simulink model "robot_linear_model"  (R2024b)
settings: Solver=VariableStepAuto  StartTime=0.0  StopTime=10.0  RelTol=1e-3
model workspace (MAT data in the model file):
  pitchd = Simulink.Parameter
  pitchd.Value = 1
  pitchd.Complexity = 'real'
  pitchd.Dimensions = [1 1]
  pitchd.DataType = 'auto'
  yawd = Simulink.Parameter
  yawd.Value = 1
  yawd.Complexity = 'real'
  yawd.Dimensions = [1 1]
  yawd.DataType = 'auto'
values from neighbouring files (symbols this model uses):
  A = [0   1.0000        0        0 ... (first row only)    [invgui.m]    (also in p1.m = 14; p2.m = 14; robot.m = [0 1 0 0; robot_cascade.m = [ 0, 1, 0, 0)
  B = [0; 1.8182; 0; 4.5455]    [invgui.m]    (also in p1.m = 18; p2.m = 18; robot.m = B ./ R; robot_cascade.m = B ./ r_wheel)
  C_xt = eye(4)    [robot.m]    (also in robot_cascade.m; robot_linear.m; robot_lqr.m)
  D_xt = [0;0;0;0]    [robot.m]    (also in robot_cascade.m; robot_linear.m; robot_lqr.m)
  Km = 0.212207    [robot.m]    (also in robot_cascade.m = 16.1290322581; robot_linear.m; robot_lqr.m)
  n = 18.75    [robot.m]    (also in robot_cascade.m; robot_linear.m; robot_lqr.m)
  r_wheel = 0.04    [robot_cascade.m]    (also in robot_linear.m; robot_lqr.m)
libraries: cstblocks x8, slctrl_autotuning x1, slpidlib x1
settings Model: Creator=cosr3  LastModifiedBy=cosr3

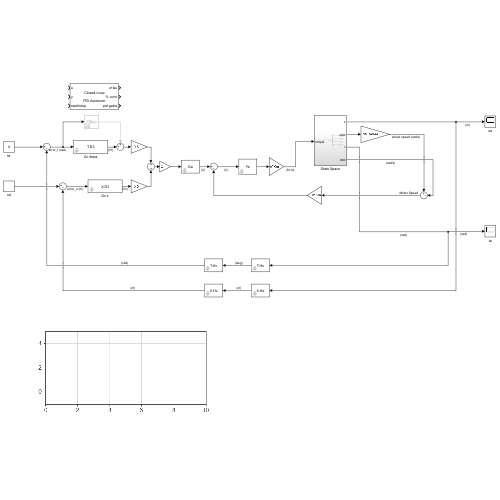
[thumbnail: Simulink's stored preview of the top-level diagram]
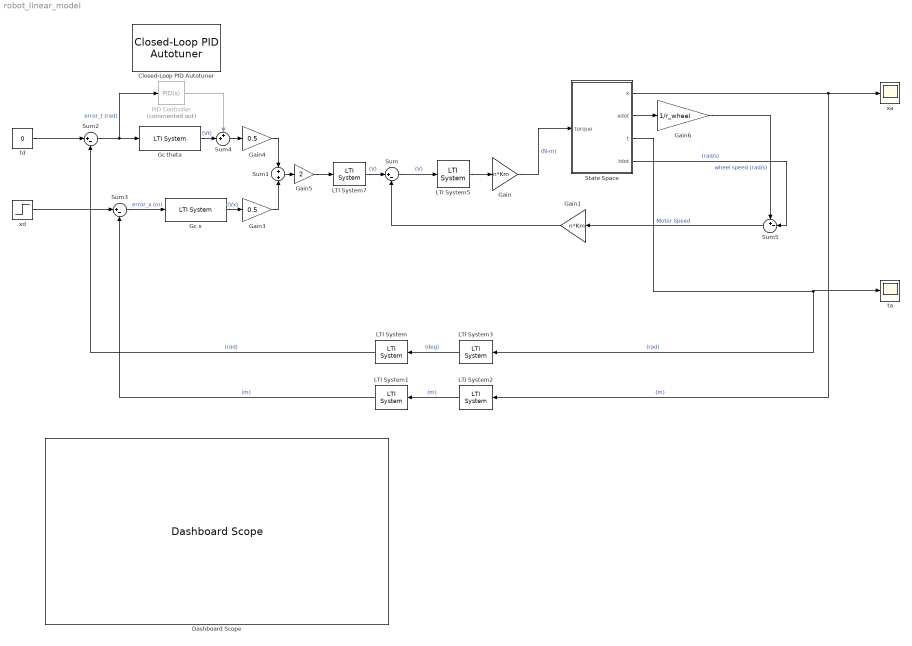
== system robot_linear_model ==
  Closed-Loop PID Autotuner : slctrl_autotuning/Closed-Loop PID Autotuner  PIDType=PI  PIDForm=Parallel  TimeDomain=discrete-time  DiscreteTs=0.1  TuningTs=0.2  UseTuningTs=off  IntegratorFormula=Forward Euler  FilterFormula=Forward Euler  ContinuousTs=0.02  Bandwidth=1  UseExternalWC=off  TargetPM=60  UseExternalPM=off  UseExternalAchievedPM=off  ExperimentMode=Superposition  PlantType=Stable  PlantSign=Positive  AmpSine=1  UseExternalAmpSine=off  UseExternalFRD=off  UseExternalU0=off  UseCompanion=off  NotDeployTuningModule=off  UsePLCCoder=off  OutputMode=control action + perturbation  BlockDataType=double  UseConnectedPID=on  blockpath=[]  tunedP=0  tunedI=0  tunedD=0  tunedN=100  tunedPM=0  EstimationWindowSize=3  UseExternalTuningParams=off  SingleMultiRateVariant=SingleSamplingRate  NumEstimationPeriods=4  NumSettlingPeriods=2  NumOfPRBSPeriod=1  PRBSSignalOrder=12  ExperimentModeVariant=VariantSuperimposed  OutputChoice=VariantCandD  ConvergenceCalcVariant=ConvSuperpositionPRBSVariant
      settings: LibrarySourceBlock=slctrlblks/Autotuning/Closed-Loop PID Autotuner
  Dashboard Scope : DashboardScope  TimeSpan=10  Ymin=-1  Ymax=5  ScaleAtStop=off
  Gain : Gain  Gain=n*Km
  Gain1 : Gain  Gain=n*Km
  Gain3 : Gain  Gain=0.5
  Gain4 : Gain  Gain=0.5
  Gain5 : Gain  Gain=2
  Gain6 : Gain  Gain=1/r_wheel
  Gc theta : cstblocks/LTI System  sys=T.D3  IC=[]  PadeOrder=0
  Gc x : cstblocks/LTI System  sys=X.D3  IC=[]  PadeOrder=0
  LTI System : cstblocks/LTI System  sys=T.Hc  IC=[]  PadeOrder=0
  LTI System1 : cstblocks/LTI System  sys=X.Hc  IC=[]  PadeOrder=0
  LTI System2 : cstblocks/LTI System  sys=X.Hs  IC=[]  PadeOrder=0
  LTI System3 : cstblocks/LTI System  sys=T.Hs  IC=[]  PadeOrder=0
  LTI System5 : cstblocks/LTI System  sys=Ye  IC=[]  PadeOrder=0
  LTI System7 : cstblocks/LTI System  sys=Ga  IC=[]  PadeOrder=0
  PID Controller : slpidlib/PID Controller  Commented=on  Controller=PID  Form=Parallel  TimeDomain=Continuous-time  UseExternalTs=off  SampleTime=-1  IntegratorMethod=Forward Euler  FilterMethod=Forward Euler  ControllerParametersSource=internal  P=5649337.82323438  I=717739936.401578  UseKiTs=off  D=8228.40688518288  UseExternalDerivativeSource=off  N=201848.584101947  UseFilter=on  TunerSelectOption=Transfer Function Based (PID Tuner App)  InitialConditionSource=internal  InitialConditionForIntegrator=0  InitialConditionForFilter=0  DifferentiatorICPrevScaledInput=0  ExternalReset=none  TrackingMode=off  Kt=1  LimitOutput=off  SatLimitsSource=internal  UpperSaturationLimit=inf  LowerSaturationLimit=-inf  LinearizeAsGain=on  AntiWindupMode=none  Kb=1  LimitIntegrator=off  UpperIntegratorSaturationLimit=inf  LowerIntegratorSaturationLimit=-inf  POutMin=[]  POutMax=[]  IOutMin=[]  IOutMax=[]  DOutMin=[]  DOutMax=[]  NOutMin=[]  NOutMax=[]  SumOutMin=[]  SumOutMax=[]  SaturationOutMin=[]  SaturationOutMax=[]  PParamMin=[]  PParamMax=[]  IParamMin=[]  IParamMax=[]  DParamMin=[]  DParamMax=[]  NParamMin=[]  NParamMax=[]  KbParamMin=[]  KbParamMax=[]  KtParamMin=[]  KtParamMax=[]  KbOutMin=[]  KbOutMax=[]  KtOutMin=[]  KtOutMax=[]  IntegratorOutMin=[]  IntegratorOutMax=[]  FilterOutMin=[]  FilterOutMax=[]  SumI1OutMin=[]  SumI1OutMax=[]  SumI2OutMin=[]  SumI2OutMax=[]  SumI3OutMin=[]  SumI3OutMax=[]  SumI4OutMin=[]  SumI4OutMax=[]  SumDOutMin=[]  SumDOutMax=[]  DifferentiatorOutMin=[]  DifferentiatorOutMax=[]  FilterDiffOutCoefMin=[]  FilterDiffOutCoefMax=[]  ReciprocalOutMin=[]  ReciprocalOutMax=[]  SumDenOutMin=[]  SumDenOutMax=[]  SumNumOutMin=[]  SumNumOutMax=[]  DivideOutMin=[]  DivideOutMax=[]  UdiffTsProdOutMin=[]  UdiffTsProdOutMax=[]  NTsProdOutMin=[]  NTsProdOutMax=[]  UintegralTsProdOutMin=[]  UintegralTsProdOutMax=[]  UngainTsProdOutMin=[]  UngainTsProdOutMax=[]  ClampingZeroOutDataTypeStr=Inherit: Inherit via back propagation  ClampingZeroOutMin=[]  ClampingZeroOutMax=[]  FilterDenConstantOutDataTypeStr=Inherit: Inherit via back propagation  FilterDenConstantOutMin=[]  FilterDenConstantOutMax=[]  PCopyOutDataTypeStr=Inherit: Inherit via back propagation  PCopyOutMin=[]  PCopyOutMax=[]  NCopyOutDataTypeStr=Inherit: Inherit via back propagation  NCopyOutMin=[]  NCopyOutMax=[]  IntegratorContinuousStateAttributes=''  IntegratorStateMustResolveToSignalObject=off  IntegratorRTWStateStorageClass=Auto  FilterContinuousStateAttributes=''  FilterStateMustResolveToSignalObject=off  FilterRTWStateStorageClass=Auto  ParallelPVariant=InternalParameters  IdealPVariant=Disabled  IVariant=InternalParameters  DVariant=InternalParameters  IntegratorVariant=Continuous  SatVariant=Disabled  AWVariant=Passthrough  PCopyVariant=Disabled  TRVariant=Disabled  FdbkBlocksVariant=Forward  IdealPFdbkVariant=Disabled  SatFdbkVariant=Disabled  DerivativeFilterVariant=ContFilter  NVariant=InternalParameters  NCopyVariant=Disabled  FilterICVariant=InternalICsFilter  IntegratorICVariant=InternalICs  ExternalResetVariant=Disabled  TRSumVariant=Passthrough  SumFdbkVariant=Disabled  SumVariant=Sum_PID  TsampFilterVariant=InternalTs  TsampNgainVariant=Passthrough  TsampIntegralVariant=Disabled_SignalSpec  ExternalSaturationOutDataTypeStr=Inherit: Same as second input  DerivativeSourceVariant=ErrorSignal  PreIntVariant=InternalPreInt
  State Space : Subsystem
  Sum : Sum  Inputs=|+-
  Sum1 : Sum
  Sum2 : Sum  Inputs=|+-
  Sum3 : Sum  Inputs=|+-
  Sum4 : Sum  Inputs=++|
  Sum5 : Sum  Inputs=+-|
  ta : Scope
  td : Constant  Value=0
  xa : Scope
  xd : Step  SampleTime=0
  wires:
  LTI System5/1 -> Gain/1
  Gain/1 -> State Space/1(torque)  "(N-m)"
  LTI System3/1 -> LTI System/1  "(deg)"
  LTI System2/1 -> LTI System1/1  "(m)"
  Sum/1 -> LTI System5/1  "(V)"
  Gain1/1 -> Sum/2
  LTI System7/1 -> Sum/1  "(V)"
  Gain4/1 -> Sum1/1
  Gain3/1 -> Sum1/2
  Gc theta/1 -> Sum4/2  "(Vt)"
  Gc x/1 -> Gain3/1  "(Vx)"
  Sum3/1 -> Gc x/1  "error_x (m)"
  Sum2/1 -> PID Controller/1, Gc theta/1  "error_t (rad)"
  td/1 -> Sum2/1
  xd/1 -> Sum3/1
  LTI System/1 -> Sum2/2  "(rad)"
  LTI System1/1 -> Sum3/2  "(m)"
  Sum1/1 -> Gain5/1
  Gain5/1 -> LTI System7/1
  State Space/1(x) -> LTI System2/1, xa/1  "(m)"
  State Space/3(t) -> LTI System3/1, ta/1  "(rad)"
  State Space/2(xdot) -> Gain6/1
  Sum5/1 -> Gain1/1  "Motor Speed"
  State Space/4(tdot) -> Sum5/2  "(rad/s)"
  Gain6/1 -> Sum5/1  "wheel speed (rad/s)"
  Sum4/1 -> Gain4/1
  PID Controller/1 -> Sum4/1

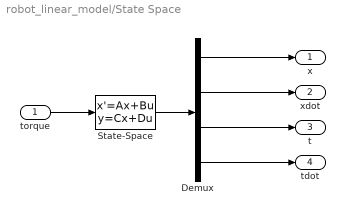
== system robot_linear_model/State Space ==
  torque : Inport
  Demux : Demux
  State-Space : StateSpace  A=A  B=B  C=C_xt  D=D_xt  InitialCondition=0
  x : Outport
  xdot : Outport  Port=2
  t : Outport  Port=3
  tdot : Outport  Port=4
  wires:
  Demux/1 -> x/1
  State-Space/1 -> Demux/1
  Demux/4 -> tdot/1
  Demux/2 -> xdot/1
  torque/1 -> State-Space/1
  Demux/3 -> t/1
